simulink model "FloatingPointIIR_DFormII"  (R2023a)
settings: Solver=VariableStepAuto  StartTime=0.0  StopTime=500  RelTol=1e-3
PreLoadFcn:
  | FloatingPointIIR_DFormII_PreLoadFcn
InitFcn:
  | xlIIRFilterResponse;
undefined symbols (not defined in the file): DEN2, DEN3, Fs, NUM1, NUM3, scale, xlIIRFilterResponse
libraries: hdlBasic x22, hdlUtilities x1, vmcUtilities x1
settings Model: Creator=viswanad  LastModifiedBy=robg
settings SolverCC: AlgebraicLoopSolver=TrustRegion
settings DataIOCC: ReturnWorkspaceOutputs=off
settings DebuggingCC: UnconnectedInputMsg=warning  UnconnectedOutputMsg=warning  UnconnectedLineMsg=warning  ArithmeticOperatorsInVariantConditions=warning
settings ModelReferenceCC: EnableRefExpFcnMdlSchedulingChecks=on
settings SFSimCC: SimUseLocalCustomCode=off  CustomCodeUndefinedFunction=UseInterfaceOnly
settings RTWCC: RTWUseLocalCustomCode=off  DLArmComputeVersion=19.05
settings CodeAppCC: StateflowObjectComments=on

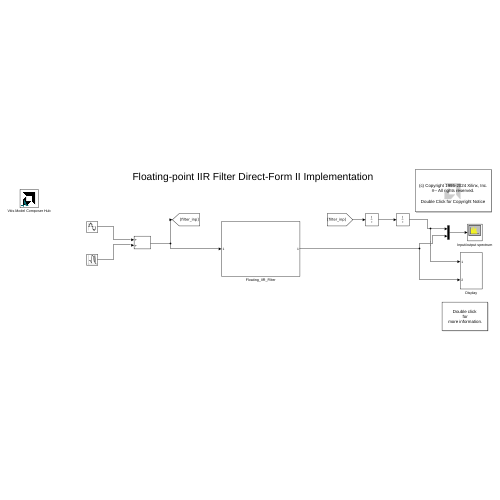
[thumbnail: Simulink's stored preview of the top-level diagram]
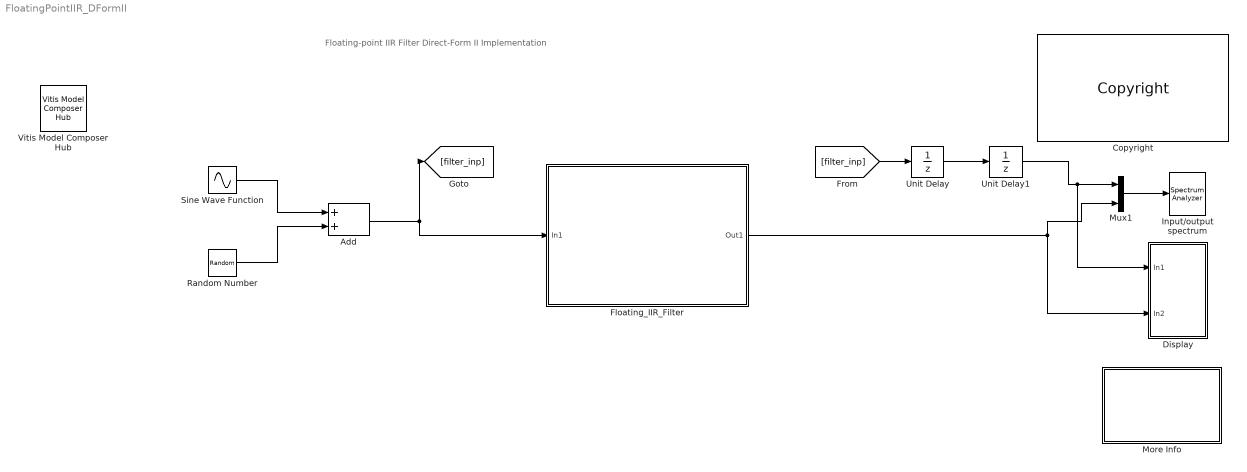
== system FloatingPointIIR_DFormII ==
  note: Floating-point IIR Filter Direct-Form II Implementation
  Add : Sum
  Copyright : hdlUtilities/Copyright  copyrighttext="Copyright (c) 2024  by  Xilinx, Inc. All rights reserved.<br><br>This file contains proprietary, confidential information of Xilinx, Inc., is distributed under license from Xilinx, Inc., and may be used, copied and/or disclosed only pursuant to the terms of a valid license agreement with Xilinx, Inc. Xilinx hereby grants you a license to use this file solely for design, simulation, implementation and creation of design files limited to Xilinx devices or technologies. Use with non-Xilinx devices or technologies is expressly prohibited and immediately terminates your license unless covered by a separate agreement.<br><br>Xilinx is providing this design, code, or information \"as-is\" solely for use in developing programs and solutions for Xilinx devices, with no obligation on the part of Xilinx to provide support. By providing this design, code, or information as one possible implementation of this feature, application or standard, Xilinx is making no representation that this implementation is free from any claims of infringement. You are responsible for obtaining any rights you may require for your implementation. Xilinx expressly disclaims any warranty whatsoever with respect to the adequacy of the implementation, including but not limited to any warranties or representations that this implementation is free from claims of infringement, implied warranties of merchantability or fitness for a particular purpose.<br><br>Xilinx products are not intended for use in life support appliances, devices, or systems. Use in such applications is expressly prohibited.<br><br>Any modifications that are made to the Source Code are done at the user's sole risk and will be unsupported.<br><br>This copyright and support notice must be retained as part of this text at all times. (c) Copyright 1995-2024 Xilinx, Inc. All rights reserved."  block_type=copyright
  Display : Subsystem
  Floating_IIR_Filter : Subsystem
  Input/output spectrum : SpectrumAnalyzer  WindowPosition=[821 389 437 231]  Visible=on  SpectrumType=Power density  Method=Welch  SampleRate=200  PlotAsTwoSidedSpectrum=off  RBWSource=Property  RBW=0.586524024  FFTLength=128  Span=100  CenterFrequency=50  StartFrequency=0  StopFrequency=100  AveragingMethod=Exponential  YLabel=Magnitude  YLimits=[-114.1297,9.8544]  ChannelNames="[\"\"]"  DefaultConfigurationName=spbscopes.SpectrumAnalyzerBlockCfg
  More Info : Subsystem
      mask Display: disp('Double click\n for\n more information.')
  Mux1 : Mux  Inputs=2
  Random Number : RandomNumber  Variance=10  SampleTime=1/(Fs)
  Sine Wave Function : Sin  Frequency=2*3.14*5000  SampleTime=1/(Fs)
  Unit Delay : UnitDelay  SampleTime=-1  HasFrameUpgradeWarning=on
  Unit Delay1 : UnitDelay  SampleTime=-1  HasFrameUpgradeWarning=on
  Vitis Model Composer Hub : vmcUtilities/Vitis Model Composer Hub  Tag=genX  CodeGeneration=off  StartColumn=1  NumberOfColumns=1  TargetDirectory=./code  exportDesign=off  analyzeDesign=off  validateDesignOnHw=off  ExportType=System Generator  IpVendor=xilinx.com  IpLibrary=hls  IpVersion=1.0  IpHWLanguage=Verilog  AieCompilerOptions={}  AieSimulatorOptions={}  CreateTestbench=off  TestbenchStackSize=10  RunRtlSim=off  RunCSim=off  RunAieSim=off  AieSimTimeout=50000  RunAieSimProfiling=off  LaunchVitisAnalyzer=off  PlotOutput=off  RunX86Sim=off  X86SimTimeout=10  GenHwImage=off  GenLibadfXo=off  GenHwValidationCode=off  PlatformType=Not Specified  HwSystemType=Baremetal  HwValidationTarget=hw  ProjDevice=xcku11p-ffva1156-1-e  ProjDevicePart=xcku11p-ffva1156-1-e  SamplePeriod=-1  ClockFrequency=200  DataPathParallelism=1  xilinxfamily=kintexuplus  part=xcku11p  speed=-1-e  package=ffva1156  directory=./netlist  testbench=off  incr_netlist=off  synthesis_tool=Vivado  clock_wrapper=Clock Enables  dbl_ovrd=According to Block Masks  dcm_input_clock_period=10  sysclk_period=10  simulink_period=1/(scale*Fs)  eval_field=0  IPInfoJsonString="{\"HDLSubsystem\":{\"SubsystemName\":\"Floating_IIR_Filter\",\"IPName\":\"Floating_IIR_Filter\",\"IPLibrary\":\"VMC\",\"IPVendor\":\"User Company\",\"IPVersion\":\"1.0\"}}"  LogFileName=''  NThreads=4
  wires:
  Add/1 -> Floating_IIR_Filter/1(In1), [filter_inp]
  Random Number/1 -> Add/2
  Unit Delay/1 -> Unit Delay1/1
  Sine Wave Function/1 -> Add/1
  Mux1/1 -> Input/output spectrum/1
  Unit Delay1/1 -> Mux1/1, Display/1(In1)
  [filter_inp] -> Unit Delay/1
  Floating_IIR_Filter/1(Out1) -> Display/2(In2), Mux1/2

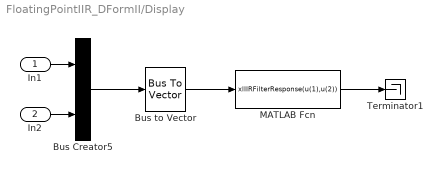
== system FloatingPointIIR_DFormII/Display ==
  In1 : Inport
  In2 : Inport  Port=2
  Bus Creator5 : BusCreator  Inputs=2
  Bus to Vector : BusToVector
  MATLAB Fcn : MATLABFcn  MATLABFcn=xlIIRFilterResponse(u(1),u(2))
  Terminator1 : Terminator
  wires:
  MATLAB Fcn/1 -> Terminator1/1
  Bus to Vector/1 -> MATLAB Fcn/1
  Bus Creator5/1 -> Bus to Vector/1
  In1/1 -> Bus Creator5/1
  In2/1 -> Bus Creator5/2

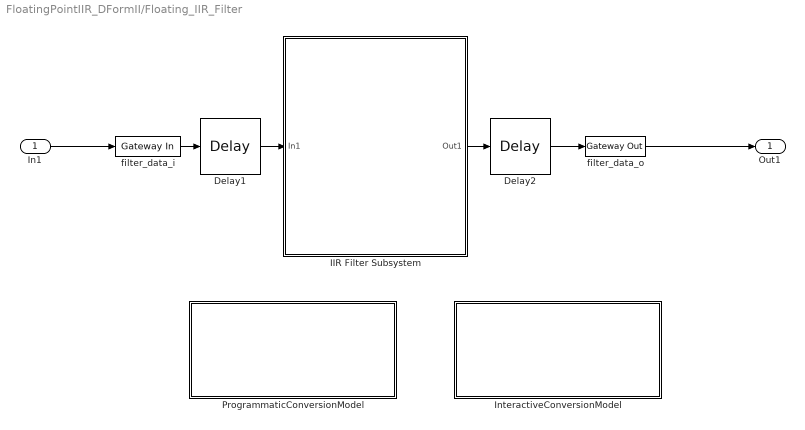
== system FloatingPointIIR_DFormII/Floating_IIR_Filter ==
  In1 : Inport
  Delay1 : hdlBasic/Delay  rst=off  en=off  latency=1  reg_retiming=off  XmcBlockStatus=1  maskContainerNames=group1  block_type=delay  block_config=sysgen:Delay_config
  Delay2 : hdlBasic/Delay  rst=off  en=off  latency=1  reg_retiming=off  XmcBlockStatus=1  maskContainerNames=group1  block_type=delay  block_config=sysgen:Delay_config
  IIR Filter Subsystem : Subsystem
  InteractiveConversionModel : Subsystem
      settings: OpenFcn=xlConvertModel_I();
      mask Display: disp('Double click\n  to\n  switch between\n  Fixed-point and Floating-point\n  interactively');
  ProgrammaticConversionModel : Subsystem
      settings: OpenFcn=xlConvertModel_P();
      mask Display: disp('Double click\n  to\n  switch between\n  Fixed-point and Floating-point\n  programmatically');
  filter_data_i : hdlBasic/Gateway In  gui_display_data_type=Floating-point  arith_type=Floating-point  n_bits=32  bin_pt=24  preci_type=Custom  exp_width=6  frac_width=9  rows=1  columns=1  quantization="Round  (unbiased: +/- Inf)"  overflow=Saturate  period=1/(Fs)  UseAsADC=off  ADCChannel='1'  interface=None  automatic_assignment=on  address_offset=hex2dec('00')  intf_name=''  intf_description=''  default_value=0  timing_constraint=None  locs_specified=off  LOCs={}  io_standard={}  inherit_from_input=off  hdl_port=on  XmcBlockStatus=1  maskContainerNames=group4  block_type=gatewayin  block_config=sysgen:gateway_in_config  block_width_w=590  block_height_w=620  block_width=640  block_height=850
  filter_data_o : hdlBasic/Gateway Out  inherit_from_input=off  hdl_port=on  rows=1  columns=1  UseAsDAC=off  DACChannel='1'  interface=None  automatic_assignment=on  address_offset=hex2dec('00')  intf_name=''  intf_description=''  timing_constraint=None  locs_specified=off  LOCs={}  io_standard={}  XmcBlockStatus=1  maskContainerNames=group4  block_type=gatewayout  block_config=sysgen:gateway_out_config  block_width_w=590  block_height_w=620  block_width=620  block_height=750
  Out1 : Outport
  wires:
  IIR Filter Subsystem/1(Out1) -> Delay2/1
  filter_data_i/1 -> Delay1/1
  Delay2/1 -> filter_data_o/1
  In1/1 -> filter_data_i/1
  Delay1/1 -> IIR Filter Subsystem/1(In1)
  filter_data_o/1 -> Out1/1

== system FloatingPointIIR_DFormII/More Info ==
  note: Floating-point IIR Filter Direct-Form II Implementation
  note: This design is a model for Direct Form II realization of a second-order IIR Filter (Peaking Filter).
      |
      | The design shows Sysgen's capability to switch between Floating point and Fixed point data.
      |
      | The same design can be modified to a Fixed-point model -
      |         a) Programmatically, using the 'ConversionModel' switch present at the top-level or
      |         b) Manually, by configuring different blocks in the system (a brief description available at the top-level)
      |
      | It can be noticed from the plotted filter-reponses, using a Floating-point system (Custom precision, Exponent-width=6, Fraction-width=9) it
      | achieves a  much better filter-response with less-than-half the total-bitwidth, when compared to the Fixed-point model (Number of bits = 32,
      | Binary point = 24).
      |
      | Implementation notes:
      |
      | For Floating-point system:
      | - Input precision ('Arithmetic type', 'Number of bits' and 'Binary point') at the GatewayIn and Constant block-GUIs should be same.
      | - Output precision at the Addsub and Multiplier blocks should be selected as 'Full' precision.
      |
      | For Fixed-point system:
      | -  Output precision ('Output type', 'Number of bits' and 'Binary point') at the Addsub and Multiplier block-GUIs should be specified explicitly,
      |     by selecting 'User defined' precision.
      |
      | The operating clock frequency for the top-level design as shown is 48KHz and input signal-frequency is 5KHz and SNR being ~ -13dB.
      |
      | At the top-level system, a counter is added to create multi-cycle paths. The counter is running at the highest rate and this forces
      | System Generator to create a CE for the IIR logic which is running at a multiple of  the FPGA clock rate.

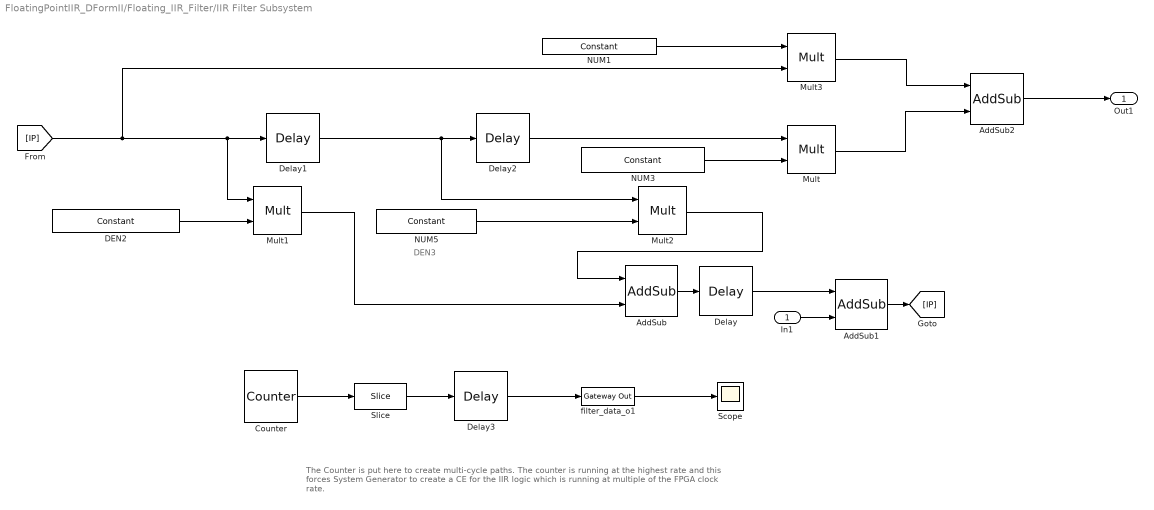
== system FloatingPointIIR_DFormII/Floating_IIR_Filter/IIR Filter Subsystem ==
  note: DEN3
  note: The Counter is put here to create multi-cycle paths. The counter is running at the highest rate
      | and this forces System Generator  to create a CE for the IIR logic which is running at multiple of  the
      | FPGA clock rate.
  In1 : Inport
  AddSub : hdlBasic/AddSub  mode=Addition  use_carryin=off  use_carryout=off  en=off  latency=0  precision=Full  arith_type="Signed  (2's comp)"  n_bits=32  bin_pt=24  quantization=Truncate  overflow=Wrap  use_behavioral_HDL=off  hw_selection=DSP48  pipelined=off  XmcBlockStatus=1  maskContainerNames=tabcontainer1  block_type=addsub  block_config=sysgen:Addsub_config
  AddSub1 : hdlBasic/AddSub  mode=Addition  use_carryin=off  use_carryout=off  en=off  latency=0  precision=Full  arith_type="Signed  (2's comp)"  n_bits=32  bin_pt=24  quantization=Truncate  overflow=Wrap  use_behavioral_HDL=off  hw_selection=DSP48  pipelined=off  XmcBlockStatus=1  maskContainerNames=tabcontainer1  block_type=addsub  block_config=sysgen:Addsub_config
  AddSub2 : hdlBasic/AddSub  mode=Addition  use_carryin=off  use_carryout=off  en=off  latency=0  precision=Full  arith_type="Signed  (2's comp)"  n_bits=32  bin_pt=24  quantization=Truncate  overflow=Wrap  use_behavioral_HDL=off  hw_selection=DSP48  pipelined=off  XmcBlockStatus=1  maskContainerNames=tabcontainer1  block_type=addsub  block_config=sysgen:Addsub_config
  Counter : hdlBasic/Counter  cnt_type=Free running  cnt_to=Inf  operation=Up  start_count=0  cnt_by_val=1  arith_type=Unsigned  n_bits=4  bin_pt=0  load_pin=off  rst=off  en=off  explicit_period=Explicit  period=1/(scale*Fs)  use_behavioral_HDL=off  implementation=Fabric  XmcBlockStatus=1  maskContainerNames=group1  block_type=counter  block_config=sysgen:Counter_config  block_width=531  block_height=1023
  DEN2 : hdlBasic/Constant  const=DEN2  gui_display_data_type=Floating-point  arith_type=Floating-point  n_bits=32  bin_pt=24  preci_type=Custom  exp_width=6  frac_width=9  explicit_period=on  period=1/(Fs)  XmcBlockStatus=1  maskContainerNames=tabcontainer1  block_type=constant  block_config=sysgen:Constant_config
  Delay{,1..3} (4 alike) : hdlBasic/Delay  rst=off  en=off  latency=1  reg_retiming=off  XmcBlockStatus=1  maskContainerNames=group1  block_type=delay  block_config=sysgen:Delay_config
  Mult{,1..3} (4 alike) : hdlBasic/Mult  precision=Full  arith_type="Signed  (2's comp)"  n_bits=32  bin_pt=24  quantization=Truncate  overflow=Wrap  en=off  latency=0  opt_float=off  fp_mult_usage=No Usage  use_behavioral_HDL=off  opt=Speed  use_embedded=on  optimum_pipeline=off  pipeline=on  use_rpm=on  placement_style=Triangular  XmcBlockStatus=1  maskContainerNames=group1  block_type=mult  block_config=sysgen:Mult_config  block_width=598  block_height=876
  NUM1 : hdlBasic/Constant  const=NUM1  gui_display_data_type=Floating-point  arith_type=Floating-point  n_bits=32  bin_pt=24  preci_type=Custom  exp_width=6  frac_width=9  explicit_period=on  period=1/(Fs)  XmcBlockStatus=1  maskContainerNames=tabcontainer1  block_type=constant  block_config=sysgen:Constant_config
  NUM3 : hdlBasic/Constant  const=NUM3  gui_display_data_type=Floating-point  arith_type=Floating-point  n_bits=32  bin_pt=24  preci_type=Custom  exp_width=6  frac_width=9  explicit_period=on  period=1/(Fs)  XmcBlockStatus=1  maskContainerNames=tabcontainer1  block_type=constant  block_config=sysgen:Constant_config
  NUM5 : hdlBasic/Constant  const=DEN3  gui_display_data_type=Floating-point  arith_type=Floating-point  n_bits=32  bin_pt=24  preci_type=Custom  exp_width=6  frac_width=9  explicit_period=on  period=1/(Fs)  XmcBlockStatus=1  maskContainerNames=tabcontainer1  block_type=constant  block_config=sysgen:Constant_config
  Scope : Scope
  Slice : hdlBasic/Slice  nbits=4  boolean_output=off  mode=Upper Bit Location + Width  bit1=0  base1=MSB of Input  bit0=0  base0=LSB of Input  XmcBlockStatus=1  maskContainerNames=group1  block_type=slice  block_config=sysgen:Slice_config
  filter_data_o1 : hdlBasic/Gateway Out  inherit_from_input=off  hdl_port=off  rows=1  columns=1  UseAsDAC=off  DACChannel='1'  interface=None  automatic_assignment=on  address_offset=hex2dec('00')  intf_name=''  intf_description=''  timing_constraint=None  locs_specified=off  LOCs={}  io_standard={}  XmcBlockStatus=1  maskContainerNames=group4  block_type=gatewayout  block_config=sysgen:gateway_out_config  block_width_w=590  block_height_w=620  block_width=620  block_height=750
  Out1 : Outport  VectorParamsAs1DForOutWhenUnconnected=off
  wires:
  Delay1/1 -> Mult2/1, Delay2/1
  NUM3/1 -> Mult/2
  DEN2/1 -> Mult1/2
  NUM5/1 -> Mult2/2
  Mult1/1 -> AddSub/2
  Mult2/1 -> AddSub/1
  NUM1/1 -> Mult3/1
  Mult3/1 -> AddSub2/1
  Mult/1 -> AddSub2/2
  [IP] -> Mult3/2, Delay1/1, Mult1/1
  AddSub2/1 -> Out1/1
  AddSub1/1 -> [IP]
  AddSub/1 -> Delay/1
  In1/1 -> AddSub1/2
  Delay/1 -> AddSub1/1
  Delay2/1 -> Mult/1
  Counter/1 -> Slice/1
  filter_data_o1/1 -> Scope/1
  Slice/1 -> Delay3/1
  Delay3/1 -> filter_data_o1/1

== system FloatingPointIIR_DFormII/Floating_IIR_Filter/InteractiveConversionModel ==

== system FloatingPointIIR_DFormII/Floating_IIR_Filter/ProgrammaticConversionModel ==
